simulink model "TST_Rail_MonMeUn"  (R2016b)
settings: Solver=FixedStepDiscrete  StartTime=0.0  StopTime=simTime  FixedStep=sampleTime  RelTol=1e-3
values from neighbouring files (symbols this model uses):
  testCase = 1    [initTST_Rail_MonMeUn_001.m]    (also in initTST_Rail_MonMeUn_002.m = 2; initTST_Rail_MonMeUn_003.m = 3; initTST_Rail_MonMeUn_004.m = 4; initTST_Rail_MonMeUn_005.m = 5)
libraries: simulink x91, UnitTest_Lib x81
(part 2 of 5)

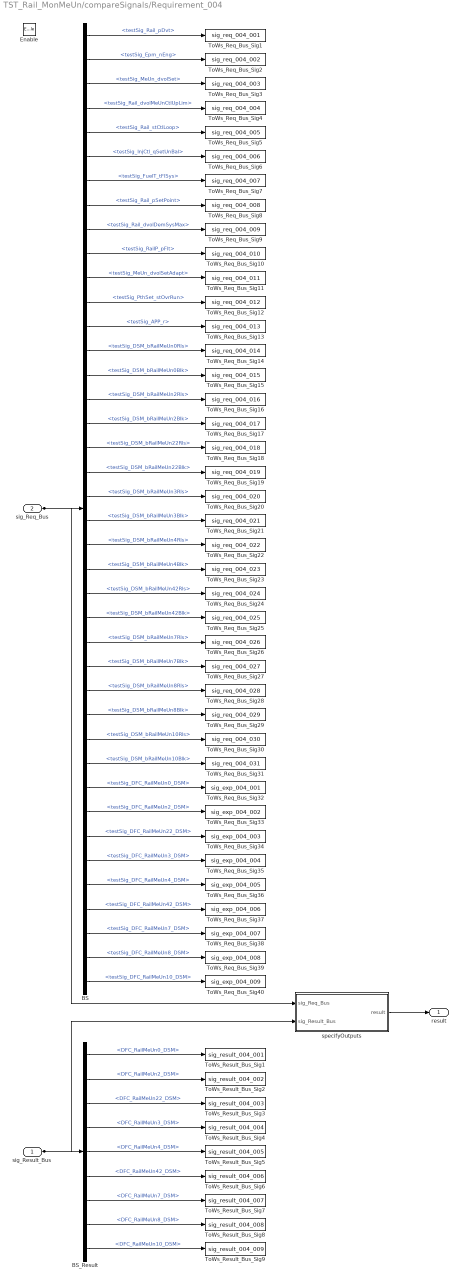
== system TST_Rail_MonMeUn/compareSignals/Requirement_004 ==
  sig_Result_Bus : Inport
  sig_Req_Bus : Inport  Port=2
  Enable : EnablePort
  BS : BusSelector  OutputSignals=testSig_Rail_pDvt,testSig_Epm_nEng,testSig_MeUn_dvolSet,testSig_Rail_dvolMeUnCtlUpLim,testSig_Rail_stCtlLoop,testSig_InjCtl_qSetUnBal,testSig_FuelT_tFlSys,testSig_Rail_pSetPoint,testSig_Rail_dvolDemSysMax,testSig_RailP_pFlt,testSig_MeUn_dvolSetAdapt,testSig_PthSet_stOvrRun,testSig_APP_r,testSig_DSM_bRailMeUn0Rls,testSig_DSM_bRailMeUn0Blk,testSig_DSM_bRailMeUn2Rls,testSig_DSM_bRailMeUn2Blk,testSig_DSM_bRailMeUn22Rls,testSig_DSM_bRailMeUn22Blk,testSig_DSM_bRailMeUn3Rls,testSig_DSM_bRailMeUn3Blk,testSig_DSM_bRailMeUn4Rls,testSig_DSM_bRailMeUn4Blk,testSig_DSM_bRailMeUn42Rls,testSig_DSM_bRailMeUn42Blk,testSig_DSM_bRailMeUn7Rls,testSig_DSM_bRailMeUn7Blk,testSig_DSM_bRailMeUn8Rls,testSig_DSM_bRailMeUn8Blk,testSig_DSM_bRailMeUn10Rls,testSig_DSM_bRailMeUn10Blk,testSig_DFC_RailMeUn0_DSM,testSig_DFC_RailMeUn2_DSM,testSig_DFC_RailMeUn22_DSM,testSig_DFC_RailMeUn3_DSM,testSig_DFC_RailMeUn4_DSM,testSig_DFC_RailMeUn42_DSM,testSig_DFC_RailMeUn7_DSM,testSig_DFC_RailMeUn8_DSM,testSig_DFC_RailMeUn10_DSM
  BS_Result : BusSelector  OutputSignals=DFC_RailMeUn0_DSM,DFC_RailMeUn2_DSM,DFC_RailMeUn22_DSM,DFC_RailMeUn3_DSM,DFC_RailMeUn4_DSM,DFC_RailMeUn42_DSM,DFC_RailMeUn7_DSM,DFC_RailMeUn8_DSM,DFC_RailMeUn10_DSM
  ToWs_Req_Bus_Sig1 : ToWorkspace  VariableName=sig_req_004_001  SaveFormat=Structure With Time
  ToWs_Req_Bus_Sig10 : ToWorkspace  VariableName=sig_req_004_010  SaveFormat=Structure With Time
  ToWs_Req_Bus_Sig11 : ToWorkspace  VariableName=sig_req_004_011  SaveFormat=Structure With Time
  ToWs_Req_Bus_Sig12 : ToWorkspace  VariableName=sig_req_004_012  SaveFormat=Structure With Time
  ToWs_Req_Bus_Sig13 : ToWorkspace  VariableName=sig_req_004_013  SaveFormat=Structure With Time
  ToWs_Req_Bus_Sig14 : ToWorkspace  VariableName=sig_req_004_014  SaveFormat=Structure With Time
  ToWs_Req_Bus_Sig15 : ToWorkspace  VariableName=sig_req_004_015  SaveFormat=Structure With Time
  ToWs_Req_Bus_Sig16 : ToWorkspace  VariableName=sig_req_004_016  SaveFormat=Structure With Time
  ToWs_Req_Bus_Sig17 : ToWorkspace  VariableName=sig_req_004_017  SaveFormat=Structure With Time
  ToWs_Req_Bus_Sig18 : ToWorkspace  VariableName=sig_req_004_018  SaveFormat=Structure With Time
  ToWs_Req_Bus_Sig19 : ToWorkspace  VariableName=sig_req_004_019  SaveFormat=Structure With Time
  ToWs_Req_Bus_Sig2 : ToWorkspace  VariableName=sig_req_004_002  SaveFormat=Structure With Time
  ToWs_Req_Bus_Sig20 : ToWorkspace  VariableName=sig_req_004_020  SaveFormat=Structure With Time
  ToWs_Req_Bus_Sig21 : ToWorkspace  VariableName=sig_req_004_021  SaveFormat=Structure With Time
  ToWs_Req_Bus_Sig22 : ToWorkspace  VariableName=sig_req_004_022  SaveFormat=Structure With Time
  ToWs_Req_Bus_Sig23 : ToWorkspace  VariableName=sig_req_004_023  SaveFormat=Structure With Time
  ToWs_Req_Bus_Sig24 : ToWorkspace  VariableName=sig_req_004_024  SaveFormat=Structure With Time
  ToWs_Req_Bus_Sig25 : ToWorkspace  VariableName=sig_req_004_025  SaveFormat=Structure With Time
  ToWs_Req_Bus_Sig26 : ToWorkspace  VariableName=sig_req_004_026  SaveFormat=Structure With Time
  ToWs_Req_Bus_Sig27 : ToWorkspace  VariableName=sig_req_004_027  SaveFormat=Structure With Time
  ToWs_Req_Bus_Sig28 : ToWorkspace  VariableName=sig_req_004_028  SaveFormat=Structure With Time
  ToWs_Req_Bus_Sig29 : ToWorkspace  VariableName=sig_req_004_029  SaveFormat=Structure With Time
  ToWs_Req_Bus_Sig3 : ToWorkspace  VariableName=sig_req_004_003  SaveFormat=Structure With Time
  ToWs_Req_Bus_Sig30 : ToWorkspace  VariableName=sig_req_004_030  SaveFormat=Structure With Time
  ToWs_Req_Bus_Sig31 : ToWorkspace  VariableName=sig_req_004_031  SaveFormat=Structure With Time
  ToWs_Req_Bus_Sig32 : ToWorkspace  VariableName=sig_exp_004_001  SaveFormat=Structure With Time
  ToWs_Req_Bus_Sig33 : ToWorkspace  VariableName=sig_exp_004_002  SaveFormat=Structure With Time
  ToWs_Req_Bus_Sig34 : ToWorkspace  VariableName=sig_exp_004_003  SaveFormat=Structure With Time
  ToWs_Req_Bus_Sig35 : ToWorkspace  VariableName=sig_exp_004_004  SaveFormat=Structure With Time
  ToWs_Req_Bus_Sig36 : ToWorkspace  VariableName=sig_exp_004_005  SaveFormat=Structure With Time
  ToWs_Req_Bus_Sig37 : ToWorkspace  VariableName=sig_exp_004_006  SaveFormat=Structure With Time
  ToWs_Req_Bus_Sig38 : ToWorkspace  VariableName=sig_exp_004_007  SaveFormat=Structure With Time
  ToWs_Req_Bus_Sig39 : ToWorkspace  VariableName=sig_exp_004_008  SaveFormat=Structure With Time
  ToWs_Req_Bus_Sig4 : ToWorkspace  VariableName=sig_req_004_004  SaveFormat=Structure With Time
  ToWs_Req_Bus_Sig40 : ToWorkspace  VariableName=sig_exp_004_009  SaveFormat=Structure With Time
  ToWs_Req_Bus_Sig5 : ToWorkspace  VariableName=sig_req_004_005  SaveFormat=Structure With Time
  ToWs_Req_Bus_Sig6 : ToWorkspace  VariableName=sig_req_004_006  SaveFormat=Structure With Time
  ToWs_Req_Bus_Sig7 : ToWorkspace  VariableName=sig_req_004_007  SaveFormat=Structure With Time
  ToWs_Req_Bus_Sig8 : ToWorkspace  VariableName=sig_req_004_008  SaveFormat=Structure With Time
  ToWs_Req_Bus_Sig9 : ToWorkspace  VariableName=sig_req_004_009  SaveFormat=Structure With Time
  ToWs_Result_Bus_Sig1 : ToWorkspace  VariableName=sig_result_004_001  SaveFormat=Structure With Time
  ToWs_Result_Bus_Sig2 : ToWorkspace  VariableName=sig_result_004_002  SaveFormat=Structure With Time
  ToWs_Result_Bus_Sig3 : ToWorkspace  VariableName=sig_result_004_003  SaveFormat=Structure With Time
  ToWs_Result_Bus_Sig4 : ToWorkspace  VariableName=sig_result_004_004  SaveFormat=Structure With Time
  ToWs_Result_Bus_Sig5 : ToWorkspace  VariableName=sig_result_004_005  SaveFormat=Structure With Time
  ToWs_Result_Bus_Sig6 : ToWorkspace  VariableName=sig_result_004_006  SaveFormat=Structure With Time
  ToWs_Result_Bus_Sig7 : ToWorkspace  VariableName=sig_result_004_007  SaveFormat=Structure With Time
  ToWs_Result_Bus_Sig8 : ToWorkspace  VariableName=sig_result_004_008  SaveFormat=Structure With Time
  ToWs_Result_Bus_Sig9 : ToWorkspace  VariableName=sig_result_004_009  SaveFormat=Structure With Time
  specifyOutputs : Subsystem
  result : Outport
  wires:
  sig_Req_Bus/1 -> BS/1, specifyOutputs/1(sig_Req_Bus)
  BS/1 -> ToWs_Req_Bus_Sig1/1  "<testSig_Rail_pDvt>"
  BS/2 -> ToWs_Req_Bus_Sig2/1  "<testSig_Epm_nEng>"
  BS/3 -> ToWs_Req_Bus_Sig3/1  "<testSig_MeUn_dvolSet>"
  BS/4 -> ToWs_Req_Bus_Sig4/1  "<testSig_Rail_dvolMeUnCtlUpLim>"
  BS/5 -> ToWs_Req_Bus_Sig5/1  "<testSig_Rail_stCtlLoop>"
  BS/6 -> ToWs_Req_Bus_Sig6/1  "<testSig_InjCtl_qSetUnBal>"
  BS/7 -> ToWs_Req_Bus_Sig7/1  "<testSig_FuelT_tFlSys>"
  BS/8 -> ToWs_Req_Bus_Sig8/1  "<testSig_Rail_pSetPoint>"
  BS/9 -> ToWs_Req_Bus_Sig9/1  "<testSig_Rail_dvolDemSysMax>"
  BS/10 -> ToWs_Req_Bus_Sig10/1  "<testSig_RailP_pFlt>"
  BS/11 -> ToWs_Req_Bus_Sig11/1  "<testSig_MeUn_dvolSetAdapt>"
  BS/12 -> ToWs_Req_Bus_Sig12/1  "<testSig_PthSet_stOvrRun>"
  BS/13 -> ToWs_Req_Bus_Sig13/1  "<testSig_APP_r>"
  BS/14 -> ToWs_Req_Bus_Sig14/1  "<testSig_DSM_bRailMeUn0Rls>"
  BS/15 -> ToWs_Req_Bus_Sig15/1  "<testSig_DSM_bRailMeUn0Blk>"
  BS/16 -> ToWs_Req_Bus_Sig16/1  "<testSig_DSM_bRailMeUn2Rls>"
  BS/17 -> ToWs_Req_Bus_Sig17/1  "<testSig_DSM_bRailMeUn2Blk>"
  BS/18 -> ToWs_Req_Bus_Sig18/1  "<testSig_DSM_bRailMeUn22Rls>"
  BS/19 -> ToWs_Req_Bus_Sig19/1  "<testSig_DSM_bRailMeUn22Blk>"
  BS/20 -> ToWs_Req_Bus_Sig20/1  "<testSig_DSM_bRailMeUn3Rls>"
  BS/21 -> ToWs_Req_Bus_Sig21/1  "<testSig_DSM_bRailMeUn3Blk>"
  BS/22 -> ToWs_Req_Bus_Sig22/1  "<testSig_DSM_bRailMeUn4Rls>"
  BS/23 -> ToWs_Req_Bus_Sig23/1  "<testSig_DSM_bRailMeUn4Blk>"
  BS/24 -> ToWs_Req_Bus_Sig24/1  "<testSig_DSM_bRailMeUn42Rls>"
  BS/25 -> ToWs_Req_Bus_Sig25/1  "<testSig_DSM_bRailMeUn42Blk>"
  BS/26 -> ToWs_Req_Bus_Sig26/1  "<testSig_DSM_bRailMeUn7Rls>"
  BS/27 -> ToWs_Req_Bus_Sig27/1  "<testSig_DSM_bRailMeUn7Blk>"
  BS/28 -> ToWs_Req_Bus_Sig28/1  "<testSig_DSM_bRailMeUn8Rls>"
  BS/29 -> ToWs_Req_Bus_Sig29/1  "<testSig_DSM_bRailMeUn8Blk>"
  BS/30 -> ToWs_Req_Bus_Sig30/1  "<testSig_DSM_bRailMeUn10Rls>"
  BS/31 -> ToWs_Req_Bus_Sig31/1  "<testSig_DSM_bRailMeUn10Blk>"
  BS/32 -> ToWs_Req_Bus_Sig32/1  "<testSig_DFC_RailMeUn0_DSM>"
  BS/33 -> ToWs_Req_Bus_Sig33/1  "<testSig_DFC_RailMeUn2_DSM>"
  BS/34 -> ToWs_Req_Bus_Sig34/1  "<testSig_DFC_RailMeUn22_DSM>"
  BS/35 -> ToWs_Req_Bus_Sig35/1  "<testSig_DFC_RailMeUn3_DSM>"
  BS/36 -> ToWs_Req_Bus_Sig36/1  "<testSig_DFC_RailMeUn4_DSM>"
  BS/37 -> ToWs_Req_Bus_Sig37/1  "<testSig_DFC_RailMeUn42_DSM>"
  BS/38 -> ToWs_Req_Bus_Sig38/1  "<testSig_DFC_RailMeUn7_DSM>"
  BS/39 -> ToWs_Req_Bus_Sig39/1  "<testSig_DFC_RailMeUn8_DSM>"
  BS/40 -> ToWs_Req_Bus_Sig40/1  "<testSig_DFC_RailMeUn10_DSM>"
  sig_Result_Bus/1 -> BS_Result/1, specifyOutputs/2(sig_Result_Bus)
  BS_Result/1 -> ToWs_Result_Bus_Sig1/1  "<DFC_RailMeUn0_DSM>"
  BS_Result/2 -> ToWs_Result_Bus_Sig2/1  "<DFC_RailMeUn2_DSM>"
  BS_Result/3 -> ToWs_Result_Bus_Sig3/1  "<DFC_RailMeUn22_DSM>"
  BS_Result/4 -> ToWs_Result_Bus_Sig4/1  "<DFC_RailMeUn3_DSM>"
  BS_Result/5 -> ToWs_Result_Bus_Sig5/1  "<DFC_RailMeUn4_DSM>"
  BS_Result/6 -> ToWs_Result_Bus_Sig6/1  "<DFC_RailMeUn42_DSM>"
  BS_Result/7 -> ToWs_Result_Bus_Sig7/1  "<DFC_RailMeUn7_DSM>"
  BS_Result/8 -> ToWs_Result_Bus_Sig8/1  "<DFC_RailMeUn8_DSM>"
  BS_Result/9 -> ToWs_Result_Bus_Sig9/1  "<DFC_RailMeUn10_DSM>"
  specifyOutputs/1(result) -> result/1

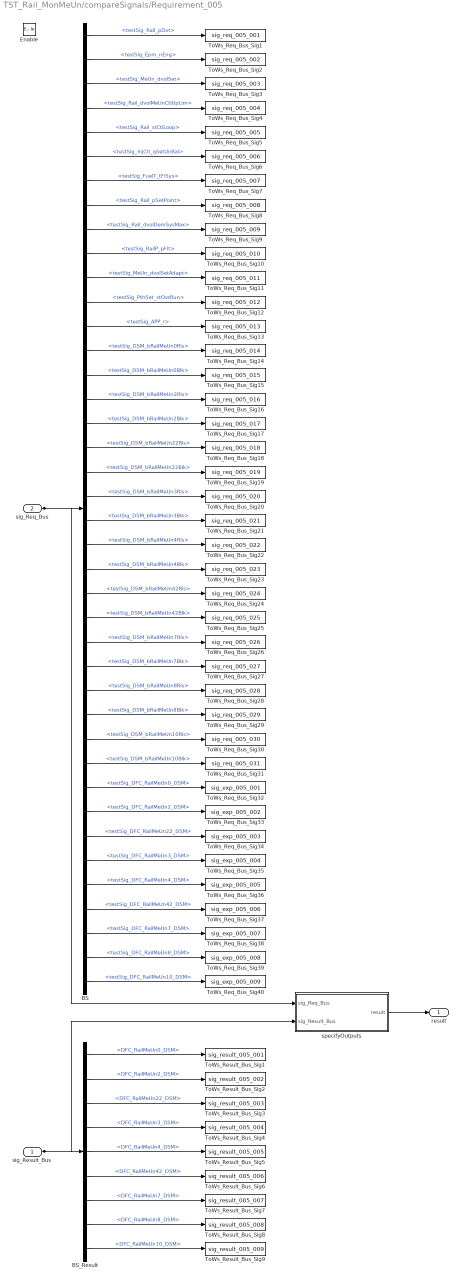
== system TST_Rail_MonMeUn/compareSignals/Requirement_005 ==
  sig_Result_Bus : Inport
  sig_Req_Bus : Inport  Port=2
  Enable : EnablePort
  BS : BusSelector  OutputSignals=testSig_Rail_pDvt,testSig_Epm_nEng,testSig_MeUn_dvolSet,testSig_Rail_dvolMeUnCtlUpLim,testSig_Rail_stCtlLoop,testSig_InjCtl_qSetUnBal,testSig_FuelT_tFlSys,testSig_Rail_pSetPoint,testSig_Rail_dvolDemSysMax,testSig_RailP_pFlt,testSig_MeUn_dvolSetAdapt,testSig_PthSet_stOvrRun,testSig_APP_r,testSig_DSM_bRailMeUn0Rls,testSig_DSM_bRailMeUn0Blk,testSig_DSM_bRailMeUn2Rls,testSig_DSM_bRailMeUn2Blk,testSig_DSM_bRailMeUn22Rls,testSig_DSM_bRailMeUn22Blk,testSig_DSM_bRailMeUn3Rls,testSig_DSM_bRailMeUn3Blk,testSig_DSM_bRailMeUn4Rls,testSig_DSM_bRailMeUn4Blk,testSig_DSM_bRailMeUn42Rls,testSig_DSM_bRailMeUn42Blk,testSig_DSM_bRailMeUn7Rls,testSig_DSM_bRailMeUn7Blk,testSig_DSM_bRailMeUn8Rls,testSig_DSM_bRailMeUn8Blk,testSig_DSM_bRailMeUn10Rls,testSig_DSM_bRailMeUn10Blk,testSig_DFC_RailMeUn0_DSM,testSig_DFC_RailMeUn2_DSM,testSig_DFC_RailMeUn22_DSM,testSig_DFC_RailMeUn3_DSM,testSig_DFC_RailMeUn4_DSM,testSig_DFC_RailMeUn42_DSM,testSig_DFC_RailMeUn7_DSM,testSig_DFC_RailMeUn8_DSM,testSig_DFC_RailMeUn10_DSM
  BS_Result : BusSelector  OutputSignals=DFC_RailMeUn0_DSM,DFC_RailMeUn2_DSM,DFC_RailMeUn22_DSM,DFC_RailMeUn3_DSM,DFC_RailMeUn4_DSM,DFC_RailMeUn42_DSM,DFC_RailMeUn7_DSM,DFC_RailMeUn8_DSM,DFC_RailMeUn10_DSM
  ToWs_Req_Bus_Sig1 : ToWorkspace  VariableName=sig_req_005_001  SaveFormat=Structure With Time
  ToWs_Req_Bus_Sig10 : ToWorkspace  VariableName=sig_req_005_010  SaveFormat=Structure With Time
  ToWs_Req_Bus_Sig11 : ToWorkspace  VariableName=sig_req_005_011  SaveFormat=Structure With Time
  ToWs_Req_Bus_Sig12 : ToWorkspace  VariableName=sig_req_005_012  SaveFormat=Structure With Time
  ToWs_Req_Bus_Sig13 : ToWorkspace  VariableName=sig_req_005_013  SaveFormat=Structure With Time
  ToWs_Req_Bus_Sig14 : ToWorkspace  VariableName=sig_req_005_014  SaveFormat=Structure With Time
  ToWs_Req_Bus_Sig15 : ToWorkspace  VariableName=sig_req_005_015  SaveFormat=Structure With Time
  ToWs_Req_Bus_Sig16 : ToWorkspace  VariableName=sig_req_005_016  SaveFormat=Structure With Time
  ToWs_Req_Bus_Sig17 : ToWorkspace  VariableName=sig_req_005_017  SaveFormat=Structure With Time
  ToWs_Req_Bus_Sig18 : ToWorkspace  VariableName=sig_req_005_018  SaveFormat=Structure With Time
  ToWs_Req_Bus_Sig19 : ToWorkspace  VariableName=sig_req_005_019  SaveFormat=Structure With Time
  ToWs_Req_Bus_Sig2 : ToWorkspace  VariableName=sig_req_005_002  SaveFormat=Structure With Time
  ToWs_Req_Bus_Sig20 : ToWorkspace  VariableName=sig_req_005_020  SaveFormat=Structure With Time
  ToWs_Req_Bus_Sig21 : ToWorkspace  VariableName=sig_req_005_021  SaveFormat=Structure With Time
  ToWs_Req_Bus_Sig22 : ToWorkspace  VariableName=sig_req_005_022  SaveFormat=Structure With Time
  ToWs_Req_Bus_Sig23 : ToWorkspace  VariableName=sig_req_005_023  SaveFormat=Structure With Time
  ToWs_Req_Bus_Sig24 : ToWorkspace  VariableName=sig_req_005_024  SaveFormat=Structure With Time
  ToWs_Req_Bus_Sig25 : ToWorkspace  VariableName=sig_req_005_025  SaveFormat=Structure With Time
  ToWs_Req_Bus_Sig26 : ToWorkspace  VariableName=sig_req_005_026  SaveFormat=Structure With Time
  ToWs_Req_Bus_Sig27 : ToWorkspace  VariableName=sig_req_005_027  SaveFormat=Structure With Time
  ToWs_Req_Bus_Sig28 : ToWorkspace  VariableName=sig_req_005_028  SaveFormat=Structure With Time
  ToWs_Req_Bus_Sig29 : ToWorkspace  VariableName=sig_req_005_029  SaveFormat=Structure With Time
  ToWs_Req_Bus_Sig3 : ToWorkspace  VariableName=sig_req_005_003  SaveFormat=Structure With Time
  ToWs_Req_Bus_Sig30 : ToWorkspace  VariableName=sig_req_005_030  SaveFormat=Structure With Time
  ToWs_Req_Bus_Sig31 : ToWorkspace  VariableName=sig_req_005_031  SaveFormat=Structure With Time
  ToWs_Req_Bus_Sig32 : ToWorkspace  VariableName=sig_exp_005_001  SaveFormat=Structure With Time
  ToWs_Req_Bus_Sig33 : ToWorkspace  VariableName=sig_exp_005_002  SaveFormat=Structure With Time
  ToWs_Req_Bus_Sig34 : ToWorkspace  VariableName=sig_exp_005_003  SaveFormat=Structure With Time
  ToWs_Req_Bus_Sig35 : ToWorkspace  VariableName=sig_exp_005_004  SaveFormat=Structure With Time
  ToWs_Req_Bus_Sig36 : ToWorkspace  VariableName=sig_exp_005_005  SaveFormat=Structure With Time
  ToWs_Req_Bus_Sig37 : ToWorkspace  VariableName=sig_exp_005_006  SaveFormat=Structure With Time
  ToWs_Req_Bus_Sig38 : ToWorkspace  VariableName=sig_exp_005_007  SaveFormat=Structure With Time
  ToWs_Req_Bus_Sig39 : ToWorkspace  VariableName=sig_exp_005_008  SaveFormat=Structure With Time
  ToWs_Req_Bus_Sig4 : ToWorkspace  VariableName=sig_req_005_004  SaveFormat=Structure With Time
  ToWs_Req_Bus_Sig40 : ToWorkspace  VariableName=sig_exp_005_009  SaveFormat=Structure With Time
  ToWs_Req_Bus_Sig5 : ToWorkspace  VariableName=sig_req_005_005  SaveFormat=Structure With Time
  ToWs_Req_Bus_Sig6 : ToWorkspace  VariableName=sig_req_005_006  SaveFormat=Structure With Time
  ToWs_Req_Bus_Sig7 : ToWorkspace  VariableName=sig_req_005_007  SaveFormat=Structure With Time
  ToWs_Req_Bus_Sig8 : ToWorkspace  VariableName=sig_req_005_008  SaveFormat=Structure With Time
  ToWs_Req_Bus_Sig9 : ToWorkspace  VariableName=sig_req_005_009  SaveFormat=Structure With Time
  ToWs_Result_Bus_Sig1 : ToWorkspace  VariableName=sig_result_005_001  SaveFormat=Structure With Time
  ToWs_Result_Bus_Sig2 : ToWorkspace  VariableName=sig_result_005_002  SaveFormat=Structure With Time
  ToWs_Result_Bus_Sig3 : ToWorkspace  VariableName=sig_result_005_003  SaveFormat=Structure With Time
  ToWs_Result_Bus_Sig4 : ToWorkspace  VariableName=sig_result_005_004  SaveFormat=Structure With Time
  ToWs_Result_Bus_Sig5 : ToWorkspace  VariableName=sig_result_005_005  SaveFormat=Structure With Time
  ToWs_Result_Bus_Sig6 : ToWorkspace  VariableName=sig_result_005_006  SaveFormat=Structure With Time
  ToWs_Result_Bus_Sig7 : ToWorkspace  VariableName=sig_result_005_007  SaveFormat=Structure With Time
  ToWs_Result_Bus_Sig8 : ToWorkspace  VariableName=sig_result_005_008  SaveFormat=Structure With Time
  ToWs_Result_Bus_Sig9 : ToWorkspace  VariableName=sig_result_005_009  SaveFormat=Structure With Time
  specifyOutputs : Subsystem
  result : Outport
  wires:
  sig_Req_Bus/1 -> BS/1, specifyOutputs/1(sig_Req_Bus)
  BS/1 -> ToWs_Req_Bus_Sig1/1  "<testSig_Rail_pDvt>"
  BS/2 -> ToWs_Req_Bus_Sig2/1  "<testSig_Epm_nEng>"
  BS/3 -> ToWs_Req_Bus_Sig3/1  "<testSig_MeUn_dvolSet>"
  BS/4 -> ToWs_Req_Bus_Sig4/1  "<testSig_Rail_dvolMeUnCtlUpLim>"
  BS/5 -> ToWs_Req_Bus_Sig5/1  "<testSig_Rail_stCtlLoop>"
  BS/6 -> ToWs_Req_Bus_Sig6/1  "<testSig_InjCtl_qSetUnBal>"
  BS/7 -> ToWs_Req_Bus_Sig7/1  "<testSig_FuelT_tFlSys>"
  BS/8 -> ToWs_Req_Bus_Sig8/1  "<testSig_Rail_pSetPoint>"
  BS/9 -> ToWs_Req_Bus_Sig9/1  "<testSig_Rail_dvolDemSysMax>"
  BS/10 -> ToWs_Req_Bus_Sig10/1  "<testSig_RailP_pFlt>"
  BS/11 -> ToWs_Req_Bus_Sig11/1  "<testSig_MeUn_dvolSetAdapt>"
  BS/12 -> ToWs_Req_Bus_Sig12/1  "<testSig_PthSet_stOvrRun>"
  BS/13 -> ToWs_Req_Bus_Sig13/1  "<testSig_APP_r>"
  BS/14 -> ToWs_Req_Bus_Sig14/1  "<testSig_DSM_bRailMeUn0Rls>"
  BS/15 -> ToWs_Req_Bus_Sig15/1  "<testSig_DSM_bRailMeUn0Blk>"
  BS/16 -> ToWs_Req_Bus_Sig16/1  "<testSig_DSM_bRailMeUn2Rls>"
  BS/17 -> ToWs_Req_Bus_Sig17/1  "<testSig_DSM_bRailMeUn2Blk>"
  BS/18 -> ToWs_Req_Bus_Sig18/1  "<testSig_DSM_bRailMeUn22Rls>"
  BS/19 -> ToWs_Req_Bus_Sig19/1  "<testSig_DSM_bRailMeUn22Blk>"
  BS/20 -> ToWs_Req_Bus_Sig20/1  "<testSig_DSM_bRailMeUn3Rls>"
  BS/21 -> ToWs_Req_Bus_Sig21/1  "<testSig_DSM_bRailMeUn3Blk>"
  BS/22 -> ToWs_Req_Bus_Sig22/1  "<testSig_DSM_bRailMeUn4Rls>"
  BS/23 -> ToWs_Req_Bus_Sig23/1  "<testSig_DSM_bRailMeUn4Blk>"
  BS/24 -> ToWs_Req_Bus_Sig24/1  "<testSig_DSM_bRailMeUn42Rls>"
  BS/25 -> ToWs_Req_Bus_Sig25/1  "<testSig_DSM_bRailMeUn42Blk>"
  BS/26 -> ToWs_Req_Bus_Sig26/1  "<testSig_DSM_bRailMeUn7Rls>"
  BS/27 -> ToWs_Req_Bus_Sig27/1  "<testSig_DSM_bRailMeUn7Blk>"
  BS/28 -> ToWs_Req_Bus_Sig28/1  "<testSig_DSM_bRailMeUn8Rls>"
  BS/29 -> ToWs_Req_Bus_Sig29/1  "<testSig_DSM_bRailMeUn8Blk>"
  BS/30 -> ToWs_Req_Bus_Sig30/1  "<testSig_DSM_bRailMeUn10Rls>"
  BS/31 -> ToWs_Req_Bus_Sig31/1  "<testSig_DSM_bRailMeUn10Blk>"
  BS/32 -> ToWs_Req_Bus_Sig32/1  "<testSig_DFC_RailMeUn0_DSM>"
  BS/33 -> ToWs_Req_Bus_Sig33/1  "<testSig_DFC_RailMeUn2_DSM>"
  BS/34 -> ToWs_Req_Bus_Sig34/1  "<testSig_DFC_RailMeUn22_DSM>"
  BS/35 -> ToWs_Req_Bus_Sig35/1  "<testSig_DFC_RailMeUn3_DSM>"
  BS/36 -> ToWs_Req_Bus_Sig36/1  "<testSig_DFC_RailMeUn4_DSM>"
  BS/37 -> ToWs_Req_Bus_Sig37/1  "<testSig_DFC_RailMeUn42_DSM>"
  BS/38 -> ToWs_Req_Bus_Sig38/1  "<testSig_DFC_RailMeUn7_DSM>"
  BS/39 -> ToWs_Req_Bus_Sig39/1  "<testSig_DFC_RailMeUn8_DSM>"
  BS/40 -> ToWs_Req_Bus_Sig40/1  "<testSig_DFC_RailMeUn10_DSM>"
  sig_Result_Bus/1 -> BS_Result/1, specifyOutputs/2(sig_Result_Bus)
  BS_Result/1 -> ToWs_Result_Bus_Sig1/1  "<DFC_RailMeUn0_DSM>"
  BS_Result/2 -> ToWs_Result_Bus_Sig2/1  "<DFC_RailMeUn2_DSM>"
  BS_Result/3 -> ToWs_Result_Bus_Sig3/1  "<DFC_RailMeUn22_DSM>"
  BS_Result/4 -> ToWs_Result_Bus_Sig4/1  "<DFC_RailMeUn3_DSM>"
  BS_Result/5 -> ToWs_Result_Bus_Sig5/1  "<DFC_RailMeUn4_DSM>"
  BS_Result/6 -> ToWs_Result_Bus_Sig6/1  "<DFC_RailMeUn42_DSM>"
  BS_Result/7 -> ToWs_Result_Bus_Sig7/1  "<DFC_RailMeUn7_DSM>"
  BS_Result/8 -> ToWs_Result_Bus_Sig8/1  "<DFC_RailMeUn8_DSM>"
  BS_Result/9 -> ToWs_Result_Bus_Sig9/1  "<DFC_RailMeUn10_DSM>"
  specifyOutputs/1(result) -> result/1

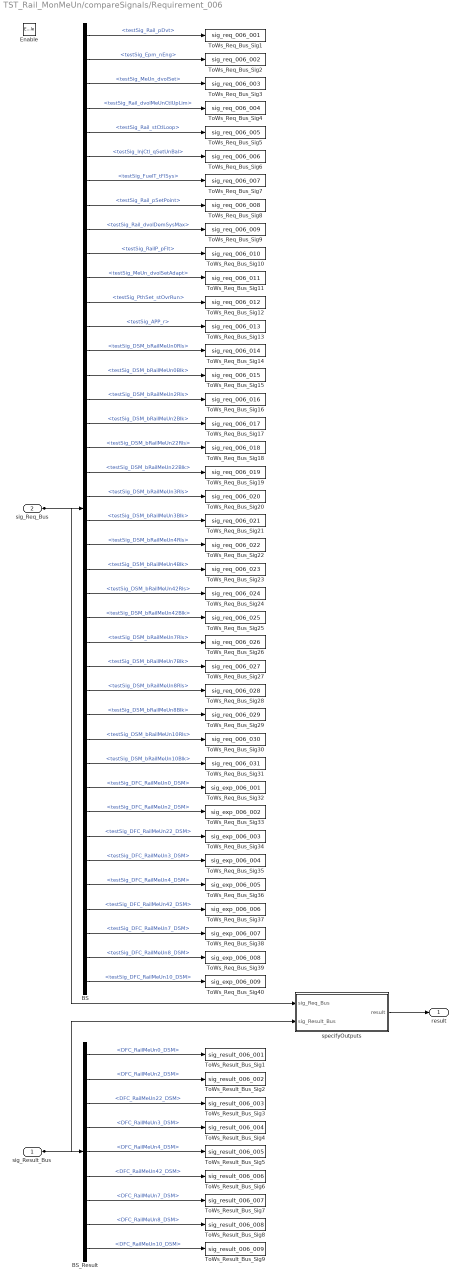
== system TST_Rail_MonMeUn/compareSignals/Requirement_006 ==
  sig_Result_Bus : Inport
  sig_Req_Bus : Inport  Port=2
  Enable : EnablePort
  BS : BusSelector  OutputSignals=testSig_Rail_pDvt,testSig_Epm_nEng,testSig_MeUn_dvolSet,testSig_Rail_dvolMeUnCtlUpLim,testSig_Rail_stCtlLoop,testSig_InjCtl_qSetUnBal,testSig_FuelT_tFlSys,testSig_Rail_pSetPoint,testSig_Rail_dvolDemSysMax,testSig_RailP_pFlt,testSig_MeUn_dvolSetAdapt,testSig_PthSet_stOvrRun,testSig_APP_r,testSig_DSM_bRailMeUn0Rls,testSig_DSM_bRailMeUn0Blk,testSig_DSM_bRailMeUn2Rls,testSig_DSM_bRailMeUn2Blk,testSig_DSM_bRailMeUn22Rls,testSig_DSM_bRailMeUn22Blk,testSig_DSM_bRailMeUn3Rls,testSig_DSM_bRailMeUn3Blk,testSig_DSM_bRailMeUn4Rls,testSig_DSM_bRailMeUn4Blk,testSig_DSM_bRailMeUn42Rls,testSig_DSM_bRailMeUn42Blk,testSig_DSM_bRailMeUn7Rls,testSig_DSM_bRailMeUn7Blk,testSig_DSM_bRailMeUn8Rls,testSig_DSM_bRailMeUn8Blk,testSig_DSM_bRailMeUn10Rls,testSig_DSM_bRailMeUn10Blk,testSig_DFC_RailMeUn0_DSM,testSig_DFC_RailMeUn2_DSM,testSig_DFC_RailMeUn22_DSM,testSig_DFC_RailMeUn3_DSM,testSig_DFC_RailMeUn4_DSM,testSig_DFC_RailMeUn42_DSM,testSig_DFC_RailMeUn7_DSM,testSig_DFC_RailMeUn8_DSM,testSig_DFC_RailMeUn10_DSM
  BS_Result : BusSelector  OutputSignals=DFC_RailMeUn0_DSM,DFC_RailMeUn2_DSM,DFC_RailMeUn22_DSM,DFC_RailMeUn3_DSM,DFC_RailMeUn4_DSM,DFC_RailMeUn42_DSM,DFC_RailMeUn7_DSM,DFC_RailMeUn8_DSM,DFC_RailMeUn10_DSM
  ToWs_Req_Bus_Sig1 : ToWorkspace  VariableName=sig_req_006_001  SaveFormat=Structure With Time
  ToWs_Req_Bus_Sig10 : ToWorkspace  VariableName=sig_req_006_010  SaveFormat=Structure With Time
  ToWs_Req_Bus_Sig11 : ToWorkspace  VariableName=sig_req_006_011  SaveFormat=Structure With Time
  ToWs_Req_Bus_Sig12 : ToWorkspace  VariableName=sig_req_006_012  SaveFormat=Structure With Time
  ToWs_Req_Bus_Sig13 : ToWorkspace  VariableName=sig_req_006_013  SaveFormat=Structure With Time
  ToWs_Req_Bus_Sig14 : ToWorkspace  VariableName=sig_req_006_014  SaveFormat=Structure With Time
  ToWs_Req_Bus_Sig15 : ToWorkspace  VariableName=sig_req_006_015  SaveFormat=Structure With Time
  ToWs_Req_Bus_Sig16 : ToWorkspace  VariableName=sig_req_006_016  SaveFormat=Structure With Time
  ToWs_Req_Bus_Sig17 : ToWorkspace  VariableName=sig_req_006_017  SaveFormat=Structure With Time
  ToWs_Req_Bus_Sig18 : ToWorkspace  VariableName=sig_req_006_018  SaveFormat=Structure With Time
  ToWs_Req_Bus_Sig19 : ToWorkspace  VariableName=sig_req_006_019  SaveFormat=Structure With Time
  ToWs_Req_Bus_Sig2 : ToWorkspace  VariableName=sig_req_006_002  SaveFormat=Structure With Time
  ToWs_Req_Bus_Sig20 : ToWorkspace  VariableName=sig_req_006_020  SaveFormat=Structure With Time
  ToWs_Req_Bus_Sig21 : ToWorkspace  VariableName=sig_req_006_021  SaveFormat=Structure With Time
  ToWs_Req_Bus_Sig22 : ToWorkspace  VariableName=sig_req_006_022  SaveFormat=Structure With Time
  ToWs_Req_Bus_Sig23 : ToWorkspace  VariableName=sig_req_006_023  SaveFormat=Structure With Time
  ToWs_Req_Bus_Sig24 : ToWorkspace  VariableName=sig_req_006_024  SaveFormat=Structure With Time
  ToWs_Req_Bus_Sig25 : ToWorkspace  VariableName=sig_req_006_025  SaveFormat=Structure With Time
  ToWs_Req_Bus_Sig26 : ToWorkspace  VariableName=sig_req_006_026  SaveFormat=Structure With Time
  ToWs_Req_Bus_Sig27 : ToWorkspace  VariableName=sig_req_006_027  SaveFormat=Structure With Time
  ToWs_Req_Bus_Sig28 : ToWorkspace  VariableName=sig_req_006_028  SaveFormat=Structure With Time
  ToWs_Req_Bus_Sig29 : ToWorkspace  VariableName=sig_req_006_029  SaveFormat=Structure With Time
  ToWs_Req_Bus_Sig3 : ToWorkspace  VariableName=sig_req_006_003  SaveFormat=Structure With Time
  ToWs_Req_Bus_Sig30 : ToWorkspace  VariableName=sig_req_006_030  SaveFormat=Structure With Time
  ToWs_Req_Bus_Sig31 : ToWorkspace  VariableName=sig_req_006_031  SaveFormat=Structure With Time
  ToWs_Req_Bus_Sig32 : ToWorkspace  VariableName=sig_exp_006_001  SaveFormat=Structure With Time
  ToWs_Req_Bus_Sig33 : ToWorkspace  VariableName=sig_exp_006_002  SaveFormat=Structure With Time
  ToWs_Req_Bus_Sig34 : ToWorkspace  VariableName=sig_exp_006_003  SaveFormat=Structure With Time
  ToWs_Req_Bus_Sig35 : ToWorkspace  VariableName=sig_exp_006_004  SaveFormat=Structure With Time
  ToWs_Req_Bus_Sig36 : ToWorkspace  VariableName=sig_exp_006_005  SaveFormat=Structure With Time
  ToWs_Req_Bus_Sig37 : ToWorkspace  VariableName=sig_exp_006_006  SaveFormat=Structure With Time
  ToWs_Req_Bus_Sig38 : ToWorkspace  VariableName=sig_exp_006_007  SaveFormat=Structure With Time
  ToWs_Req_Bus_Sig39 : ToWorkspace  VariableName=sig_exp_006_008  SaveFormat=Structure With Time
  ToWs_Req_Bus_Sig4 : ToWorkspace  VariableName=sig_req_006_004  SaveFormat=Structure With Time
  ToWs_Req_Bus_Sig40 : ToWorkspace  VariableName=sig_exp_006_009  SaveFormat=Structure With Time
  ToWs_Req_Bus_Sig5 : ToWorkspace  VariableName=sig_req_006_005  SaveFormat=Structure With Time
  ToWs_Req_Bus_Sig6 : ToWorkspace  VariableName=sig_req_006_006  SaveFormat=Structure With Time
  ToWs_Req_Bus_Sig7 : ToWorkspace  VariableName=sig_req_006_007  SaveFormat=Structure With Time
  ToWs_Req_Bus_Sig8 : ToWorkspace  VariableName=sig_req_006_008  SaveFormat=Structure With Time
  ToWs_Req_Bus_Sig9 : ToWorkspace  VariableName=sig_req_006_009  SaveFormat=Structure With Time
  ToWs_Result_Bus_Sig1 : ToWorkspace  VariableName=sig_result_006_001  SaveFormat=Structure With Time
  ToWs_Result_Bus_Sig2 : ToWorkspace  VariableName=sig_result_006_002  SaveFormat=Structure With Time
  ToWs_Result_Bus_Sig3 : ToWorkspace  VariableName=sig_result_006_003  SaveFormat=Structure With Time
  ToWs_Result_Bus_Sig4 : ToWorkspace  VariableName=sig_result_006_004  SaveFormat=Structure With Time
  ToWs_Result_Bus_Sig5 : ToWorkspace  VariableName=sig_result_006_005  SaveFormat=Structure With Time
  ToWs_Result_Bus_Sig6 : ToWorkspace  VariableName=sig_result_006_006  SaveFormat=Structure With Time
  ToWs_Result_Bus_Sig7 : ToWorkspace  VariableName=sig_result_006_007  SaveFormat=Structure With Time
  ToWs_Result_Bus_Sig8 : ToWorkspace  VariableName=sig_result_006_008  SaveFormat=Structure With Time
  ToWs_Result_Bus_Sig9 : ToWorkspace  VariableName=sig_result_006_009  SaveFormat=Structure With Time
  specifyOutputs : Subsystem
  result : Outport
  wires:
  sig_Req_Bus/1 -> BS/1, specifyOutputs/1(sig_Req_Bus)
  BS/1 -> ToWs_Req_Bus_Sig1/1  "<testSig_Rail_pDvt>"
  BS/2 -> ToWs_Req_Bus_Sig2/1  "<testSig_Epm_nEng>"
  BS/3 -> ToWs_Req_Bus_Sig3/1  "<testSig_MeUn_dvolSet>"
  BS/4 -> ToWs_Req_Bus_Sig4/1  "<testSig_Rail_dvolMeUnCtlUpLim>"
  BS/5 -> ToWs_Req_Bus_Sig5/1  "<testSig_Rail_stCtlLoop>"
  BS/6 -> ToWs_Req_Bus_Sig6/1  "<testSig_InjCtl_qSetUnBal>"
  BS/7 -> ToWs_Req_Bus_Sig7/1  "<testSig_FuelT_tFlSys>"
  BS/8 -> ToWs_Req_Bus_Sig8/1  "<testSig_Rail_pSetPoint>"
  BS/9 -> ToWs_Req_Bus_Sig9/1  "<testSig_Rail_dvolDemSysMax>"
  BS/10 -> ToWs_Req_Bus_Sig10/1  "<testSig_RailP_pFlt>"
  BS/11 -> ToWs_Req_Bus_Sig11/1  "<testSig_MeUn_dvolSetAdapt>"
  BS/12 -> ToWs_Req_Bus_Sig12/1  "<testSig_PthSet_stOvrRun>"
  BS/13 -> ToWs_Req_Bus_Sig13/1  "<testSig_APP_r>"
  BS/14 -> ToWs_Req_Bus_Sig14/1  "<testSig_DSM_bRailMeUn0Rls>"
  BS/15 -> ToWs_Req_Bus_Sig15/1  "<testSig_DSM_bRailMeUn0Blk>"
  BS/16 -> ToWs_Req_Bus_Sig16/1  "<testSig_DSM_bRailMeUn2Rls>"
  BS/17 -> ToWs_Req_Bus_Sig17/1  "<testSig_DSM_bRailMeUn2Blk>"
  BS/18 -> ToWs_Req_Bus_Sig18/1  "<testSig_DSM_bRailMeUn22Rls>"
  BS/19 -> ToWs_Req_Bus_Sig19/1  "<testSig_DSM_bRailMeUn22Blk>"
  BS/20 -> ToWs_Req_Bus_Sig20/1  "<testSig_DSM_bRailMeUn3Rls>"
  BS/21 -> ToWs_Req_Bus_Sig21/1  "<testSig_DSM_bRailMeUn3Blk>"
  BS/22 -> ToWs_Req_Bus_Sig22/1  "<testSig_DSM_bRailMeUn4Rls>"
  BS/23 -> ToWs_Req_Bus_Sig23/1  "<testSig_DSM_bRailMeUn4Blk>"
  BS/24 -> ToWs_Req_Bus_Sig24/1  "<testSig_DSM_bRailMeUn42Rls>"
  BS/25 -> ToWs_Req_Bus_Sig25/1  "<testSig_DSM_bRailMeUn42Blk>"
  BS/26 -> ToWs_Req_Bus_Sig26/1  "<testSig_DSM_bRailMeUn7Rls>"
  BS/27 -> ToWs_Req_Bus_Sig27/1  "<testSig_DSM_bRailMeUn7Blk>"
  BS/28 -> ToWs_Req_Bus_Sig28/1  "<testSig_DSM_bRailMeUn8Rls>"
  BS/29 -> ToWs_Req_Bus_Sig29/1  "<testSig_DSM_bRailMeUn8Blk>"
  BS/30 -> ToWs_Req_Bus_Sig30/1  "<testSig_DSM_bRailMeUn10Rls>"
  BS/31 -> ToWs_Req_Bus_Sig31/1  "<testSig_DSM_bRailMeUn10Blk>"
  BS/32 -> ToWs_Req_Bus_Sig32/1  "<testSig_DFC_RailMeUn0_DSM>"
  BS/33 -> ToWs_Req_Bus_Sig33/1  "<testSig_DFC_RailMeUn2_DSM>"
  BS/34 -> ToWs_Req_Bus_Sig34/1  "<testSig_DFC_RailMeUn22_DSM>"
  BS/35 -> ToWs_Req_Bus_Sig35/1  "<testSig_DFC_RailMeUn3_DSM>"
  BS/36 -> ToWs_Req_Bus_Sig36/1  "<testSig_DFC_RailMeUn4_DSM>"
  BS/37 -> ToWs_Req_Bus_Sig37/1  "<testSig_DFC_RailMeUn42_DSM>"
  BS/38 -> ToWs_Req_Bus_Sig38/1  "<testSig_DFC_RailMeUn7_DSM>"
  BS/39 -> ToWs_Req_Bus_Sig39/1  "<testSig_DFC_RailMeUn8_DSM>"
  BS/40 -> ToWs_Req_Bus_Sig40/1  "<testSig_DFC_RailMeUn10_DSM>"
  sig_Result_Bus/1 -> BS_Result/1, specifyOutputs/2(sig_Result_Bus)
  BS_Result/1 -> ToWs_Result_Bus_Sig1/1  "<DFC_RailMeUn0_DSM>"
  BS_Result/2 -> ToWs_Result_Bus_Sig2/1  "<DFC_RailMeUn2_DSM>"
  BS_Result/3 -> ToWs_Result_Bus_Sig3/1  "<DFC_RailMeUn22_DSM>"
  BS_Result/4 -> ToWs_Result_Bus_Sig4/1  "<DFC_RailMeUn3_DSM>"
  BS_Result/5 -> ToWs_Result_Bus_Sig5/1  "<DFC_RailMeUn4_DSM>"
  BS_Result/6 -> ToWs_Result_Bus_Sig6/1  "<DFC_RailMeUn42_DSM>"
  BS_Result/7 -> ToWs_Result_Bus_Sig7/1  "<DFC_RailMeUn7_DSM>"
  BS_Result/8 -> ToWs_Result_Bus_Sig8/1  "<DFC_RailMeUn8_DSM>"
  BS_Result/9 -> ToWs_Result_Bus_Sig9/1  "<DFC_RailMeUn10_DSM>"
  specifyOutputs/1(result) -> result/1

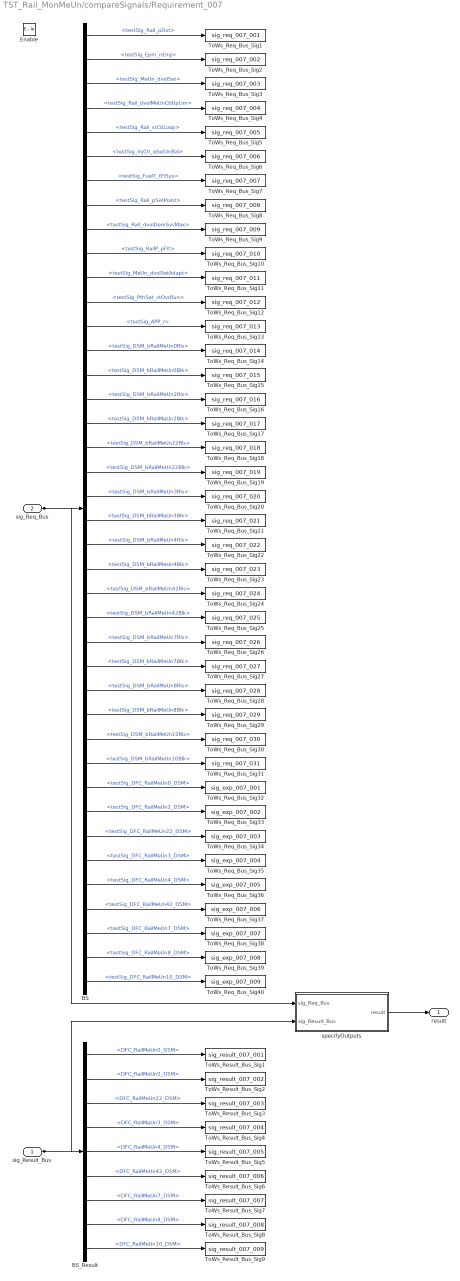
== system TST_Rail_MonMeUn/compareSignals/Requirement_007 ==
  sig_Result_Bus : Inport
  sig_Req_Bus : Inport  Port=2
  Enable : EnablePort
  BS : BusSelector  OutputSignals=testSig_Rail_pDvt,testSig_Epm_nEng,testSig_MeUn_dvolSet,testSig_Rail_dvolMeUnCtlUpLim,testSig_Rail_stCtlLoop,testSig_InjCtl_qSetUnBal,testSig_FuelT_tFlSys,testSig_Rail_pSetPoint,testSig_Rail_dvolDemSysMax,testSig_RailP_pFlt,testSig_MeUn_dvolSetAdapt,testSig_PthSet_stOvrRun,testSig_APP_r,testSig_DSM_bRailMeUn0Rls,testSig_DSM_bRailMeUn0Blk,testSig_DSM_bRailMeUn2Rls,testSig_DSM_bRailMeUn2Blk,testSig_DSM_bRailMeUn22Rls,testSig_DSM_bRailMeUn22Blk,testSig_DSM_bRailMeUn3Rls,testSig_DSM_bRailMeUn3Blk,testSig_DSM_bRailMeUn4Rls,testSig_DSM_bRailMeUn4Blk,testSig_DSM_bRailMeUn42Rls,testSig_DSM_bRailMeUn42Blk,testSig_DSM_bRailMeUn7Rls,testSig_DSM_bRailMeUn7Blk,testSig_DSM_bRailMeUn8Rls,testSig_DSM_bRailMeUn8Blk,testSig_DSM_bRailMeUn10Rls,testSig_DSM_bRailMeUn10Blk,testSig_DFC_RailMeUn0_DSM,testSig_DFC_RailMeUn2_DSM,testSig_DFC_RailMeUn22_DSM,testSig_DFC_RailMeUn3_DSM,testSig_DFC_RailMeUn4_DSM,testSig_DFC_RailMeUn42_DSM,testSig_DFC_RailMeUn7_DSM,testSig_DFC_RailMeUn8_DSM,testSig_DFC_RailMeUn10_DSM
  BS_Result : BusSelector  OutputSignals=DFC_RailMeUn0_DSM,DFC_RailMeUn2_DSM,DFC_RailMeUn22_DSM,DFC_RailMeUn3_DSM,DFC_RailMeUn4_DSM,DFC_RailMeUn42_DSM,DFC_RailMeUn7_DSM,DFC_RailMeUn8_DSM,DFC_RailMeUn10_DSM
  ToWs_Req_Bus_Sig1 : ToWorkspace  VariableName=sig_req_007_001  SaveFormat=Structure With Time
  ToWs_Req_Bus_Sig10 : ToWorkspace  VariableName=sig_req_007_010  SaveFormat=Structure With Time
  ToWs_Req_Bus_Sig11 : ToWorkspace  VariableName=sig_req_007_011  SaveFormat=Structure With Time
  ToWs_Req_Bus_Sig12 : ToWorkspace  VariableName=sig_req_007_012  SaveFormat=Structure With Time
  ToWs_Req_Bus_Sig13 : ToWorkspace  VariableName=sig_req_007_013  SaveFormat=Structure With Time
  ToWs_Req_Bus_Sig14 : ToWorkspace  VariableName=sig_req_007_014  SaveFormat=Structure With Time
  ToWs_Req_Bus_Sig15 : ToWorkspace  VariableName=sig_req_007_015  SaveFormat=Structure With Time
  ToWs_Req_Bus_Sig16 : ToWorkspace  VariableName=sig_req_007_016  SaveFormat=Structure With Time
  ToWs_Req_Bus_Sig17 : ToWorkspace  VariableName=sig_req_007_017  SaveFormat=Structure With Time
  ToWs_Req_Bus_Sig18 : ToWorkspace  VariableName=sig_req_007_018  SaveFormat=Structure With Time
  ToWs_Req_Bus_Sig19 : ToWorkspace  VariableName=sig_req_007_019  SaveFormat=Structure With Time
  ToWs_Req_Bus_Sig2 : ToWorkspace  VariableName=sig_req_007_002  SaveFormat=Structure With Time
  ToWs_Req_Bus_Sig20 : ToWorkspace  VariableName=sig_req_007_020  SaveFormat=Structure With Time
  ToWs_Req_Bus_Sig21 : ToWorkspace  VariableName=sig_req_007_021  SaveFormat=Structure With Time
  ToWs_Req_Bus_Sig22 : ToWorkspace  VariableName=sig_req_007_022  SaveFormat=Structure With Time
  ToWs_Req_Bus_Sig23 : ToWorkspace  VariableName=sig_req_007_023  SaveFormat=Structure With Time
  ToWs_Req_Bus_Sig24 : ToWorkspace  VariableName=sig_req_007_024  SaveFormat=Structure With Time
  ToWs_Req_Bus_Sig25 : ToWorkspace  VariableName=sig_req_007_025  SaveFormat=Structure With Time
  ToWs_Req_Bus_Sig26 : ToWorkspace  VariableName=sig_req_007_026  SaveFormat=Structure With Time
  ToWs_Req_Bus_Sig27 : ToWorkspace  VariableName=sig_req_007_027  SaveFormat=Structure With Time
  ToWs_Req_Bus_Sig28 : ToWorkspace  VariableName=sig_req_007_028  SaveFormat=Structure With Time
  ToWs_Req_Bus_Sig29 : ToWorkspace  VariableName=sig_req_007_029  SaveFormat=Structure With Time
  ToWs_Req_Bus_Sig3 : ToWorkspace  VariableName=sig_req_007_003  SaveFormat=Structure With Time
  ToWs_Req_Bus_Sig30 : ToWorkspace  VariableName=sig_req_007_030  SaveFormat=Structure With Time
  ToWs_Req_Bus_Sig31 : ToWorkspace  VariableName=sig_req_007_031  SaveFormat=Structure With Time
  ToWs_Req_Bus_Sig32 : ToWorkspace  VariableName=sig_exp_007_001  SaveFormat=Structure With Time
  ToWs_Req_Bus_Sig33 : ToWorkspace  VariableName=sig_exp_007_002  SaveFormat=Structure With Time
  ToWs_Req_Bus_Sig34 : ToWorkspace  VariableName=sig_exp_007_003  SaveFormat=Structure With Time
  ToWs_Req_Bus_Sig35 : ToWorkspace  VariableName=sig_exp_007_004  SaveFormat=Structure With Time
  ToWs_Req_Bus_Sig36 : ToWorkspace  VariableName=sig_exp_007_005  SaveFormat=Structure With Time
  ToWs_Req_Bus_Sig37 : ToWorkspace  VariableName=sig_exp_007_006  SaveFormat=Structure With Time
  ToWs_Req_Bus_Sig38 : ToWorkspace  VariableName=sig_exp_007_007  SaveFormat=Structure With Time
  ToWs_Req_Bus_Sig39 : ToWorkspace  VariableName=sig_exp_007_008  SaveFormat=Structure With Time
  ToWs_Req_Bus_Sig4 : ToWorkspace  VariableName=sig_req_007_004  SaveFormat=Structure With Time
  ToWs_Req_Bus_Sig40 : ToWorkspace  VariableName=sig_exp_007_009  SaveFormat=Structure With Time
  ToWs_Req_Bus_Sig5 : ToWorkspace  VariableName=sig_req_007_005  SaveFormat=Structure With Time
  ToWs_Req_Bus_Sig6 : ToWorkspace  VariableName=sig_req_007_006  SaveFormat=Structure With Time
  ToWs_Req_Bus_Sig7 : ToWorkspace  VariableName=sig_req_007_007  SaveFormat=Structure With Time
  ToWs_Req_Bus_Sig8 : ToWorkspace  VariableName=sig_req_007_008  SaveFormat=Structure With Time
  ToWs_Req_Bus_Sig9 : ToWorkspace  VariableName=sig_req_007_009  SaveFormat=Structure With Time
  ToWs_Result_Bus_Sig1 : ToWorkspace  VariableName=sig_result_007_001  SaveFormat=Structure With Time
  ToWs_Result_Bus_Sig2 : ToWorkspace  VariableName=sig_result_007_002  SaveFormat=Structure With Time
  ToWs_Result_Bus_Sig3 : ToWorkspace  VariableName=sig_result_007_003  SaveFormat=Structure With Time
  ToWs_Result_Bus_Sig4 : ToWorkspace  VariableName=sig_result_007_004  SaveFormat=Structure With Time
  ToWs_Result_Bus_Sig5 : ToWorkspace  VariableName=sig_result_007_005  SaveFormat=Structure With Time
  ToWs_Result_Bus_Sig6 : ToWorkspace  VariableName=sig_result_007_006  SaveFormat=Structure With Time
  ToWs_Result_Bus_Sig7 : ToWorkspace  VariableName=sig_result_007_007  SaveFormat=Structure With Time
  ToWs_Result_Bus_Sig8 : ToWorkspace  VariableName=sig_result_007_008  SaveFormat=Structure With Time
  ToWs_Result_Bus_Sig9 : ToWorkspace  VariableName=sig_result_007_009  SaveFormat=Structure With Time
  specifyOutputs : Subsystem
  result : Outport
  wires:
  sig_Req_Bus/1 -> BS/1, specifyOutputs/1(sig_Req_Bus)
  BS/1 -> ToWs_Req_Bus_Sig1/1  "<testSig_Rail_pDvt>"
  BS/2 -> ToWs_Req_Bus_Sig2/1  "<testSig_Epm_nEng>"
  BS/3 -> ToWs_Req_Bus_Sig3/1  "<testSig_MeUn_dvolSet>"
  BS/4 -> ToWs_Req_Bus_Sig4/1  "<testSig_Rail_dvolMeUnCtlUpLim>"
  BS/5 -> ToWs_Req_Bus_Sig5/1  "<testSig_Rail_stCtlLoop>"
  BS/6 -> ToWs_Req_Bus_Sig6/1  "<testSig_InjCtl_qSetUnBal>"
  BS/7 -> ToWs_Req_Bus_Sig7/1  "<testSig_FuelT_tFlSys>"
  BS/8 -> ToWs_Req_Bus_Sig8/1  "<testSig_Rail_pSetPoint>"
  BS/9 -> ToWs_Req_Bus_Sig9/1  "<testSig_Rail_dvolDemSysMax>"
  BS/10 -> ToWs_Req_Bus_Sig10/1  "<testSig_RailP_pFlt>"
  BS/11 -> ToWs_Req_Bus_Sig11/1  "<testSig_MeUn_dvolSetAdapt>"
  BS/12 -> ToWs_Req_Bus_Sig12/1  "<testSig_PthSet_stOvrRun>"
  BS/13 -> ToWs_Req_Bus_Sig13/1  "<testSig_APP_r>"
  BS/14 -> ToWs_Req_Bus_Sig14/1  "<testSig_DSM_bRailMeUn0Rls>"
  BS/15 -> ToWs_Req_Bus_Sig15/1  "<testSig_DSM_bRailMeUn0Blk>"
  BS/16 -> ToWs_Req_Bus_Sig16/1  "<testSig_DSM_bRailMeUn2Rls>"
  BS/17 -> ToWs_Req_Bus_Sig17/1  "<testSig_DSM_bRailMeUn2Blk>"
  BS/18 -> ToWs_Req_Bus_Sig18/1  "<testSig_DSM_bRailMeUn22Rls>"
  BS/19 -> ToWs_Req_Bus_Sig19/1  "<testSig_DSM_bRailMeUn22Blk>"
  BS/20 -> ToWs_Req_Bus_Sig20/1  "<testSig_DSM_bRailMeUn3Rls>"
  BS/21 -> ToWs_Req_Bus_Sig21/1  "<testSig_DSM_bRailMeUn3Blk>"
  BS/22 -> ToWs_Req_Bus_Sig22/1  "<testSig_DSM_bRailMeUn4Rls>"
  BS/23 -> ToWs_Req_Bus_Sig23/1  "<testSig_DSM_bRailMeUn4Blk>"
  BS/24 -> ToWs_Req_Bus_Sig24/1  "<testSig_DSM_bRailMeUn42Rls>"
  BS/25 -> ToWs_Req_Bus_Sig25/1  "<testSig_DSM_bRailMeUn42Blk>"
  BS/26 -> ToWs_Req_Bus_Sig26/1  "<testSig_DSM_bRailMeUn7Rls>"
  BS/27 -> ToWs_Req_Bus_Sig27/1  "<testSig_DSM_bRailMeUn7Blk>"
  BS/28 -> ToWs_Req_Bus_Sig28/1  "<testSig_DSM_bRailMeUn8Rls>"
  BS/29 -> ToWs_Req_Bus_Sig29/1  "<testSig_DSM_bRailMeUn8Blk>"
  BS/30 -> ToWs_Req_Bus_Sig30/1  "<testSig_DSM_bRailMeUn10Rls>"
  BS/31 -> ToWs_Req_Bus_Sig31/1  "<testSig_DSM_bRailMeUn10Blk>"
  BS/32 -> ToWs_Req_Bus_Sig32/1  "<testSig_DFC_RailMeUn0_DSM>"
  BS/33 -> ToWs_Req_Bus_Sig33/1  "<testSig_DFC_RailMeUn2_DSM>"
  BS/34 -> ToWs_Req_Bus_Sig34/1  "<testSig_DFC_RailMeUn22_DSM>"
  BS/35 -> ToWs_Req_Bus_Sig35/1  "<testSig_DFC_RailMeUn3_DSM>"
  BS/36 -> ToWs_Req_Bus_Sig36/1  "<testSig_DFC_RailMeUn4_DSM>"
  BS/37 -> ToWs_Req_Bus_Sig37/1  "<testSig_DFC_RailMeUn42_DSM>"
  BS/38 -> ToWs_Req_Bus_Sig38/1  "<testSig_DFC_RailMeUn7_DSM>"
  BS/39 -> ToWs_Req_Bus_Sig39/1  "<testSig_DFC_RailMeUn8_DSM>"
  BS/40 -> ToWs_Req_Bus_Sig40/1  "<testSig_DFC_RailMeUn10_DSM>"
  sig_Result_Bus/1 -> BS_Result/1, specifyOutputs/2(sig_Result_Bus)
  BS_Result/1 -> ToWs_Result_Bus_Sig1/1  "<DFC_RailMeUn0_DSM>"
  BS_Result/2 -> ToWs_Result_Bus_Sig2/1  "<DFC_RailMeUn2_DSM>"
  BS_Result/3 -> ToWs_Result_Bus_Sig3/1  "<DFC_RailMeUn22_DSM>"
  BS_Result/4 -> ToWs_Result_Bus_Sig4/1  "<DFC_RailMeUn3_DSM>"
  BS_Result/5 -> ToWs_Result_Bus_Sig5/1  "<DFC_RailMeUn4_DSM>"
  BS_Result/6 -> ToWs_Result_Bus_Sig6/1  "<DFC_RailMeUn42_DSM>"
  BS_Result/7 -> ToWs_Result_Bus_Sig7/1  "<DFC_RailMeUn7_DSM>"
  BS_Result/8 -> ToWs_Result_Bus_Sig8/1  "<DFC_RailMeUn8_DSM>"
  BS_Result/9 -> ToWs_Result_Bus_Sig9/1  "<DFC_RailMeUn10_DSM>"
  specifyOutputs/1(result) -> result/1

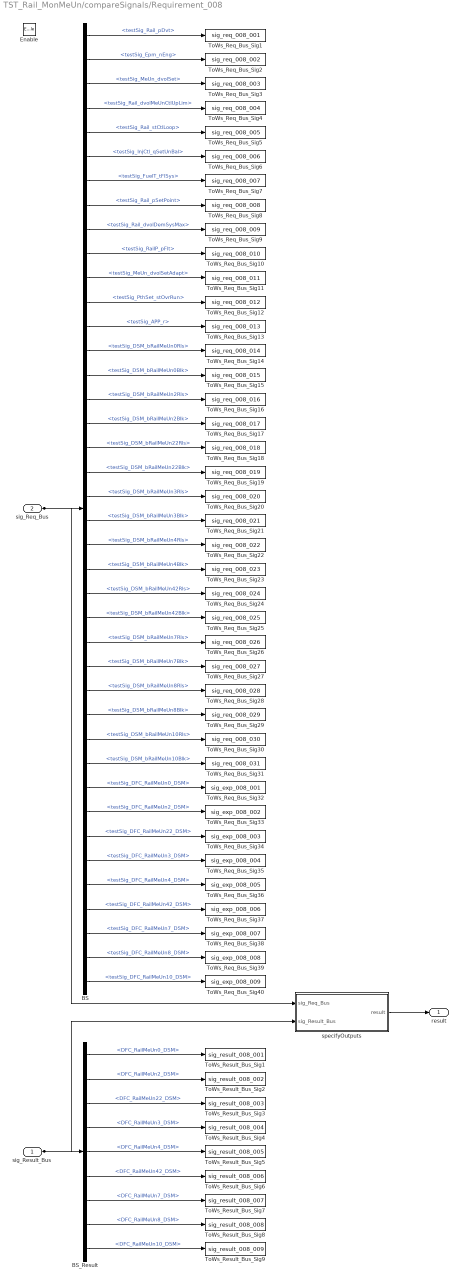
== system TST_Rail_MonMeUn/compareSignals/Requirement_008 ==
  sig_Result_Bus : Inport
  sig_Req_Bus : Inport  Port=2
  Enable : EnablePort
  BS : BusSelector  OutputSignals=testSig_Rail_pDvt,testSig_Epm_nEng,testSig_MeUn_dvolSet,testSig_Rail_dvolMeUnCtlUpLim,testSig_Rail_stCtlLoop,testSig_InjCtl_qSetUnBal,testSig_FuelT_tFlSys,testSig_Rail_pSetPoint,testSig_Rail_dvolDemSysMax,testSig_RailP_pFlt,testSig_MeUn_dvolSetAdapt,testSig_PthSet_stOvrRun,testSig_APP_r,testSig_DSM_bRailMeUn0Rls,testSig_DSM_bRailMeUn0Blk,testSig_DSM_bRailMeUn2Rls,testSig_DSM_bRailMeUn2Blk,testSig_DSM_bRailMeUn22Rls,testSig_DSM_bRailMeUn22Blk,testSig_DSM_bRailMeUn3Rls,testSig_DSM_bRailMeUn3Blk,testSig_DSM_bRailMeUn4Rls,testSig_DSM_bRailMeUn4Blk,testSig_DSM_bRailMeUn42Rls,testSig_DSM_bRailMeUn42Blk,testSig_DSM_bRailMeUn7Rls,testSig_DSM_bRailMeUn7Blk,testSig_DSM_bRailMeUn8Rls,testSig_DSM_bRailMeUn8Blk,testSig_DSM_bRailMeUn10Rls,testSig_DSM_bRailMeUn10Blk,testSig_DFC_RailMeUn0_DSM,testSig_DFC_RailMeUn2_DSM,testSig_DFC_RailMeUn22_DSM,testSig_DFC_RailMeUn3_DSM,testSig_DFC_RailMeUn4_DSM,testSig_DFC_RailMeUn42_DSM,testSig_DFC_RailMeUn7_DSM,testSig_DFC_RailMeUn8_DSM,testSig_DFC_RailMeUn10_DSM
  BS_Result : BusSelector  OutputSignals=DFC_RailMeUn0_DSM,DFC_RailMeUn2_DSM,DFC_RailMeUn22_DSM,DFC_RailMeUn3_DSM,DFC_RailMeUn4_DSM,DFC_RailMeUn42_DSM,DFC_RailMeUn7_DSM,DFC_RailMeUn8_DSM,DFC_RailMeUn10_DSM
  ToWs_Req_Bus_Sig1 : ToWorkspace  VariableName=sig_req_008_001  SaveFormat=Structure With Time
  ToWs_Req_Bus_Sig10 : ToWorkspace  VariableName=sig_req_008_010  SaveFormat=Structure With Time
  ToWs_Req_Bus_Sig11 : ToWorkspace  VariableName=sig_req_008_011  SaveFormat=Structure With Time
  ToWs_Req_Bus_Sig12 : ToWorkspace  VariableName=sig_req_008_012  SaveFormat=Structure With Time
  ToWs_Req_Bus_Sig13 : ToWorkspace  VariableName=sig_req_008_013  SaveFormat=Structure With Time
  ToWs_Req_Bus_Sig14 : ToWorkspace  VariableName=sig_req_008_014  SaveFormat=Structure With Time
  ToWs_Req_Bus_Sig15 : ToWorkspace  VariableName=sig_req_008_015  SaveFormat=Structure With Time
  ToWs_Req_Bus_Sig16 : ToWorkspace  VariableName=sig_req_008_016  SaveFormat=Structure With Time
  ToWs_Req_Bus_Sig17 : ToWorkspace  VariableName=sig_req_008_017  SaveFormat=Structure With Time
  ToWs_Req_Bus_Sig18 : ToWorkspace  VariableName=sig_req_008_018  SaveFormat=Structure With Time
  ToWs_Req_Bus_Sig19 : ToWorkspace  VariableName=sig_req_008_019  SaveFormat=Structure With Time
  ToWs_Req_Bus_Sig2 : ToWorkspace  VariableName=sig_req_008_002  SaveFormat=Structure With Time
  ToWs_Req_Bus_Sig20 : ToWorkspace  VariableName=sig_req_008_020  SaveFormat=Structure With Time
  ToWs_Req_Bus_Sig21 : ToWorkspace  VariableName=sig_req_008_021  SaveFormat=Structure With Time
  ToWs_Req_Bus_Sig22 : ToWorkspace  VariableName=sig_req_008_022  SaveFormat=Structure With Time
  ToWs_Req_Bus_Sig23 : ToWorkspace  VariableName=sig_req_008_023  SaveFormat=Structure With Time
  ToWs_Req_Bus_Sig24 : ToWorkspace  VariableName=sig_req_008_024  SaveFormat=Structure With Time
  ToWs_Req_Bus_Sig25 : ToWorkspace  VariableName=sig_req_008_025  SaveFormat=Structure With Time
  ToWs_Req_Bus_Sig26 : ToWorkspace  VariableName=sig_req_008_026  SaveFormat=Structure With Time
  ToWs_Req_Bus_Sig27 : ToWorkspace  VariableName=sig_req_008_027  SaveFormat=Structure With Time
  ToWs_Req_Bus_Sig28 : ToWorkspace  VariableName=sig_req_008_028  SaveFormat=Structure With Time
  ToWs_Req_Bus_Sig29 : ToWorkspace  VariableName=sig_req_008_029  SaveFormat=Structure With Time
  ToWs_Req_Bus_Sig3 : ToWorkspace  VariableName=sig_req_008_003  SaveFormat=Structure With Time
  ToWs_Req_Bus_Sig30 : ToWorkspace  VariableName=sig_req_008_030  SaveFormat=Structure With Time
  ToWs_Req_Bus_Sig31 : ToWorkspace  VariableName=sig_req_008_031  SaveFormat=Structure With Time
  ToWs_Req_Bus_Sig32 : ToWorkspace  VariableName=sig_exp_008_001  SaveFormat=Structure With Time
  ToWs_Req_Bus_Sig33 : ToWorkspace  VariableName=sig_exp_008_002  SaveFormat=Structure With Time
  ToWs_Req_Bus_Sig34 : ToWorkspace  VariableName=sig_exp_008_003  SaveFormat=Structure With Time
  ToWs_Req_Bus_Sig35 : ToWorkspace  VariableName=sig_exp_008_004  SaveFormat=Structure With Time
  ToWs_Req_Bus_Sig36 : ToWorkspace  VariableName=sig_exp_008_005  SaveFormat=Structure With Time
  ToWs_Req_Bus_Sig37 : ToWorkspace  VariableName=sig_exp_008_006  SaveFormat=Structure With Time
  ToWs_Req_Bus_Sig38 : ToWorkspace  VariableName=sig_exp_008_007  SaveFormat=Structure With Time
  ToWs_Req_Bus_Sig39 : ToWorkspace  VariableName=sig_exp_008_008  SaveFormat=Structure With Time
  ToWs_Req_Bus_Sig4 : ToWorkspace  VariableName=sig_req_008_004  SaveFormat=Structure With Time
  ToWs_Req_Bus_Sig40 : ToWorkspace  VariableName=sig_exp_008_009  SaveFormat=Structure With Time
  ToWs_Req_Bus_Sig5 : ToWorkspace  VariableName=sig_req_008_005  SaveFormat=Structure With Time
  ToWs_Req_Bus_Sig6 : ToWorkspace  VariableName=sig_req_008_006  SaveFormat=Structure With Time
  ToWs_Req_Bus_Sig7 : ToWorkspace  VariableName=sig_req_008_007  SaveFormat=Structure With Time
  ToWs_Req_Bus_Sig8 : ToWorkspace  VariableName=sig_req_008_008  SaveFormat=Structure With Time
  ToWs_Req_Bus_Sig9 : ToWorkspace  VariableName=sig_req_008_009  SaveFormat=Structure With Time
  ToWs_Result_Bus_Sig1 : ToWorkspace  VariableName=sig_result_008_001  SaveFormat=Structure With Time
  ToWs_Result_Bus_Sig2 : ToWorkspace  VariableName=sig_result_008_002  SaveFormat=Structure With Time
  ToWs_Result_Bus_Sig3 : ToWorkspace  VariableName=sig_result_008_003  SaveFormat=Structure With Time
  ToWs_Result_Bus_Sig4 : ToWorkspace  VariableName=sig_result_008_004  SaveFormat=Structure With Time
  ToWs_Result_Bus_Sig5 : ToWorkspace  VariableName=sig_result_008_005  SaveFormat=Structure With Time
  ToWs_Result_Bus_Sig6 : ToWorkspace  VariableName=sig_result_008_006  SaveFormat=Structure With Time
  ToWs_Result_Bus_Sig7 : ToWorkspace  VariableName=sig_result_008_007  SaveFormat=Structure With Time
  ToWs_Result_Bus_Sig8 : ToWorkspace  VariableName=sig_result_008_008  SaveFormat=Structure With Time
  ToWs_Result_Bus_Sig9 : ToWorkspace  VariableName=sig_result_008_009  SaveFormat=Structure With Time
  specifyOutputs : Subsystem
  result : Outport
  wires:
  sig_Req_Bus/1 -> BS/1, specifyOutputs/1(sig_Req_Bus)
  BS/1 -> ToWs_Req_Bus_Sig1/1  "<testSig_Rail_pDvt>"
  BS/2 -> ToWs_Req_Bus_Sig2/1  "<testSig_Epm_nEng>"
  BS/3 -> ToWs_Req_Bus_Sig3/1  "<testSig_MeUn_dvolSet>"
  BS/4 -> ToWs_Req_Bus_Sig4/1  "<testSig_Rail_dvolMeUnCtlUpLim>"
  BS/5 -> ToWs_Req_Bus_Sig5/1  "<testSig_Rail_stCtlLoop>"
  BS/6 -> ToWs_Req_Bus_Sig6/1  "<testSig_InjCtl_qSetUnBal>"
  BS/7 -> ToWs_Req_Bus_Sig7/1  "<testSig_FuelT_tFlSys>"
  BS/8 -> ToWs_Req_Bus_Sig8/1  "<testSig_Rail_pSetPoint>"
  BS/9 -> ToWs_Req_Bus_Sig9/1  "<testSig_Rail_dvolDemSysMax>"
  BS/10 -> ToWs_Req_Bus_Sig10/1  "<testSig_RailP_pFlt>"
  BS/11 -> ToWs_Req_Bus_Sig11/1  "<testSig_MeUn_dvolSetAdapt>"
  BS/12 -> ToWs_Req_Bus_Sig12/1  "<testSig_PthSet_stOvrRun>"
  BS/13 -> ToWs_Req_Bus_Sig13/1  "<testSig_APP_r>"
  BS/14 -> ToWs_Req_Bus_Sig14/1  "<testSig_DSM_bRailMeUn0Rls>"
  BS/15 -> ToWs_Req_Bus_Sig15/1  "<testSig_DSM_bRailMeUn0Blk>"
  BS/16 -> ToWs_Req_Bus_Sig16/1  "<testSig_DSM_bRailMeUn2Rls>"
  BS/17 -> ToWs_Req_Bus_Sig17/1  "<testSig_DSM_bRailMeUn2Blk>"
  BS/18 -> ToWs_Req_Bus_Sig18/1  "<testSig_DSM_bRailMeUn22Rls>"
  BS/19 -> ToWs_Req_Bus_Sig19/1  "<testSig_DSM_bRailMeUn22Blk>"
  BS/20 -> ToWs_Req_Bus_Sig20/1  "<testSig_DSM_bRailMeUn3Rls>"
  BS/21 -> ToWs_Req_Bus_Sig21/1  "<testSig_DSM_bRailMeUn3Blk>"
  BS/22 -> ToWs_Req_Bus_Sig22/1  "<testSig_DSM_bRailMeUn4Rls>"
  BS/23 -> ToWs_Req_Bus_Sig23/1  "<testSig_DSM_bRailMeUn4Blk>"
  BS/24 -> ToWs_Req_Bus_Sig24/1  "<testSig_DSM_bRailMeUn42Rls>"
  BS/25 -> ToWs_Req_Bus_Sig25/1  "<testSig_DSM_bRailMeUn42Blk>"
  BS/26 -> ToWs_Req_Bus_Sig26/1  "<testSig_DSM_bRailMeUn7Rls>"
  BS/27 -> ToWs_Req_Bus_Sig27/1  "<testSig_DSM_bRailMeUn7Blk>"
  BS/28 -> ToWs_Req_Bus_Sig28/1  "<testSig_DSM_bRailMeUn8Rls>"
  BS/29 -> ToWs_Req_Bus_Sig29/1  "<testSig_DSM_bRailMeUn8Blk>"
  BS/30 -> ToWs_Req_Bus_Sig30/1  "<testSig_DSM_bRailMeUn10Rls>"
  BS/31 -> ToWs_Req_Bus_Sig31/1  "<testSig_DSM_bRailMeUn10Blk>"
  BS/32 -> ToWs_Req_Bus_Sig32/1  "<testSig_DFC_RailMeUn0_DSM>"
  BS/33 -> ToWs_Req_Bus_Sig33/1  "<testSig_DFC_RailMeUn2_DSM>"
  BS/34 -> ToWs_Req_Bus_Sig34/1  "<testSig_DFC_RailMeUn22_DSM>"
  BS/35 -> ToWs_Req_Bus_Sig35/1  "<testSig_DFC_RailMeUn3_DSM>"
  BS/36 -> ToWs_Req_Bus_Sig36/1  "<testSig_DFC_RailMeUn4_DSM>"
  BS/37 -> ToWs_Req_Bus_Sig37/1  "<testSig_DFC_RailMeUn42_DSM>"
  BS/38 -> ToWs_Req_Bus_Sig38/1  "<testSig_DFC_RailMeUn7_DSM>"
  BS/39 -> ToWs_Req_Bus_Sig39/1  "<testSig_DFC_RailMeUn8_DSM>"
  BS/40 -> ToWs_Req_Bus_Sig40/1  "<testSig_DFC_RailMeUn10_DSM>"
  sig_Result_Bus/1 -> BS_Result/1, specifyOutputs/2(sig_Result_Bus)
  BS_Result/1 -> ToWs_Result_Bus_Sig1/1  "<DFC_RailMeUn0_DSM>"
  BS_Result/2 -> ToWs_Result_Bus_Sig2/1  "<DFC_RailMeUn2_DSM>"
  BS_Result/3 -> ToWs_Result_Bus_Sig3/1  "<DFC_RailMeUn22_DSM>"
  BS_Result/4 -> ToWs_Result_Bus_Sig4/1  "<DFC_RailMeUn3_DSM>"
  BS_Result/5 -> ToWs_Result_Bus_Sig5/1  "<DFC_RailMeUn4_DSM>"
  BS_Result/6 -> ToWs_Result_Bus_Sig6/1  "<DFC_RailMeUn42_DSM>"
  BS_Result/7 -> ToWs_Result_Bus_Sig7/1  "<DFC_RailMeUn7_DSM>"
  BS_Result/8 -> ToWs_Result_Bus_Sig8/1  "<DFC_RailMeUn8_DSM>"
  BS_Result/9 -> ToWs_Result_Bus_Sig9/1  "<DFC_RailMeUn10_DSM>"
  specifyOutputs/1(result) -> result/1
